simulink model "gps_tracking_both_allsub"  (R2018a)
settings: Solver=VariableStepAuto  StartTime=0.0  StopTime=5*16368/16367600  RelTol=1e-3
libraries: xbsIndex_r4 x171, dspsrcs4 x1
(part 1 of 2)
settings Model: Creator=zhati  LastModifiedBy=Doc_v
settings CodeAppCC: StateflowObjectComments=on
settings SimscapeCC: SimscapeNormalizeSystem=off

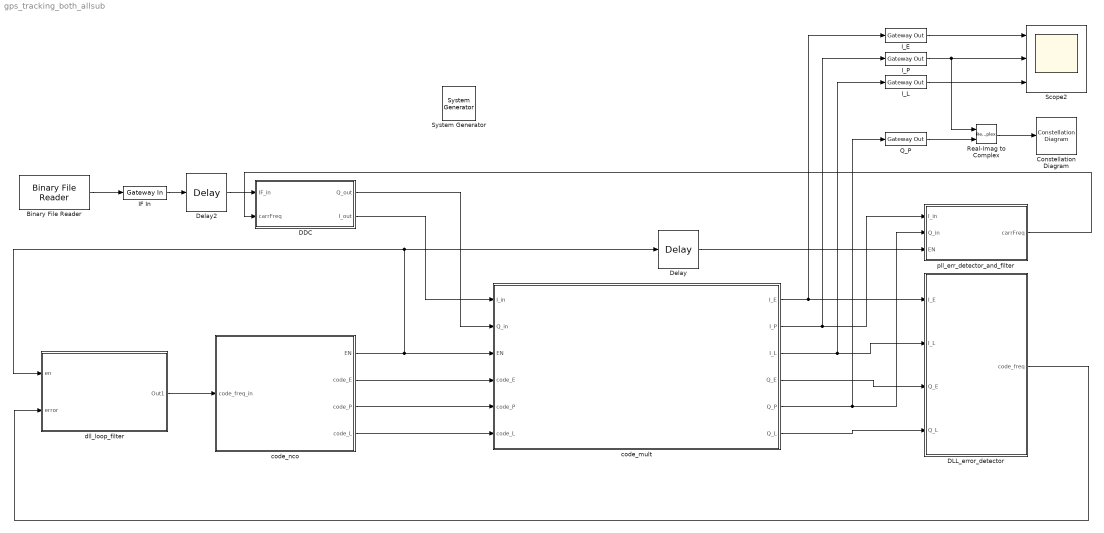
== system gps_tracking_both_allsub ==
  " I_P" : xbsIndex_r4/Gateway Out  inherit_from_input=off  hdl_port=on  rows=1  columns=1  UseAsDAC=off  DACChannel='1'  interface=None  automatic_assignment=on  address_offset=hex2dec('00')  intf_name=''  intf_description=''  timing_constraint=None  locs_specified=off  LOCs={}  io_standard={}  block_type=gatewayout
  " System Generator" : xbsIndex_r4/ System Generator  Tag=genX  xilinxfamily=kintex7  part=xc7k325t  speed=-2  package=ffg900  synthesis_tool=Vivado  clock_wrapper=Clock Enables  directory=./gps_tracking_both_allsub_hwc1  proj_type=Vivado  Synth_file=Vivado Synthesis Defaults  Impl_file=Vivado Implementation Defaults  testbench=on  simulink_period=1/16367600  sysclk_period=10  dcm_input_clock_period=10  incr_netlist=off  trim_vbits=Everywhere in SubSystem  dbl_ovrd=According to Block Masks  core_generation=According to Block Masks  run_coregen=off  deprecated_control=off  eval_field=0  block_type=sysgen
  Binary File Reader : dspsrcs4/Binary File Reader  Filename=E:\sysgen_workspace\gioveAandB_short.bin  HeaderStructure=struct([])  DataType=int8  SamplesPerFrame=1  IsDataComplex=off  NumChannels=1  OutputEOF=off  SampleTime=1/16367600  SimulateUsing=Code generation
      settings: SourceProductName=DSP System Toolbox  SourceProductBaseCode=DS
  Constellation Diagram : ConstellationDiagram
  DDC : Subsystem
  DLL_error_detector : Subsystem
  Delay : xbsIndex_r4/Delay  rst=off  infoeditControl=Selection of Reset will increase slice count due to use of real FFs and instead of SRLs  en=off  latency=1  reg_retiming=off  dbl_ovrd=off  block_type=delay
  Delay2 : xbsIndex_r4/Delay  rst=off  infoeditControl=Selection of Reset will increase slice count due to use of real FFs and instead of SRLs  en=off  latency=1312+28  reg_retiming=off  dbl_ovrd=off  block_type=delay
  IF In : xbsIndex_r4/Gateway In  gui_display_data_type=Fixed-point  arith_type="Signed  (2's comp)"  n_bits=3  bin_pt=0  preci_type=Single  exp_width=8  frac_width=24  rows=1  columns=1  quantization="Round  (unbiased: +/- Inf)"  overflow=Flag as error  period=1/16367600  UseAsADC=off  ADCChannel='1'  interface=None  automatic_assignment=on  address_offset=hex2dec('00')  intf_name=''  intf_description=''  default_value=0  timing_constraint=None  locs_specified=off  LOCs={}  io_standard={}  inherit_from_input=off  hdl_port=on  dbl_ovrd=off  block_type=gatewayin
  I_E : xbsIndex_r4/Gateway Out  inherit_from_input=off  hdl_port=on  rows=1  columns=1  UseAsDAC=off  DACChannel='1'  interface=None  automatic_assignment=on  address_offset=hex2dec('00')  intf_name=''  intf_description=''  timing_constraint=None  locs_specified=off  LOCs={}  io_standard={}  block_type=gatewayout
  I_L : xbsIndex_r4/Gateway Out  inherit_from_input=off  hdl_port=on  rows=1  columns=1  UseAsDAC=off  DACChannel='1'  interface=None  automatic_assignment=on  address_offset=hex2dec('00')  intf_name=''  intf_description=''  timing_constraint=None  locs_specified=off  LOCs={}  io_standard={}  block_type=gatewayout
  Q_P : xbsIndex_r4/Gateway Out  inherit_from_input=off  hdl_port=on  rows=1  columns=1  UseAsDAC=off  DACChannel='1'  interface=None  automatic_assignment=on  address_offset=hex2dec('00')  intf_name=''  intf_description=''  timing_constraint=None  locs_specified=off  LOCs={}  io_standard={}  block_type=gatewayout
  Real-Imag to Complex : RealImagToComplex
  Scope2 : Scope  NumInputPorts=3
  code_mult : Subsystem
  code_nco : Subsystem
  dll_loop_filter : Subsystem
  pll_err_detector_and_filter : Subsystem
  wires:
  Binary File Reader/1 -> IF In/1
  IF In/1 -> Delay2/1
  DLL_error_detector/1(code_freq) -> dll_loop_filter/2(error)
  dll_loop_filter/1(Out1) -> code_nco/1(code_freq_in)
  Delay2/1 -> DDC/1(IF_in)
  code_nco/2(code_E) -> code_mult/4(code_E)
  code_nco/3(code_P) -> code_mult/5(code_P)
  code_nco/4(code_L) -> code_mult/6(code_L)
  code_mult/1(I_E) -> I_E/1, DLL_error_detector/1(I_E)
  code_mult/3(I_L) -> I_L/1, DLL_error_detector/2(I_L)
  code_mult/4(Q_E) -> DLL_error_detector/3(Q_E)
  code_mult/6(Q_L) -> DLL_error_detector/4(Q_L)
  code_nco/1(EN) -> dll_loop_filter/1(en), Delay/1, code_mult/3(EN)
  DDC/2(I_out) -> code_mult/1(I_in)
  DDC/1(Q_out) -> code_mult/2(Q_in)
  code_mult/2(I_P) -> pll_err_detector_and_filter/1(I_in), " I_P"/1
  code_mult/5(Q_P) -> Q_P/1, pll_err_detector_and_filter/2(Q_in)
  Delay/1 -> pll_err_detector_and_filter/3(EN)
  pll_err_detector_and_filter/1(carrFreq) -> DDC/2(carrFreq)
  I_E/1 -> Scope2/1
  " I_P"/1 -> Real-Imag to Complex/1, Scope2/2
  I_L/1 -> Scope2/3
  Q_P/1 -> Real-Imag to Complex/2
  Real-Imag to Complex/1 -> Constellation Diagram/1

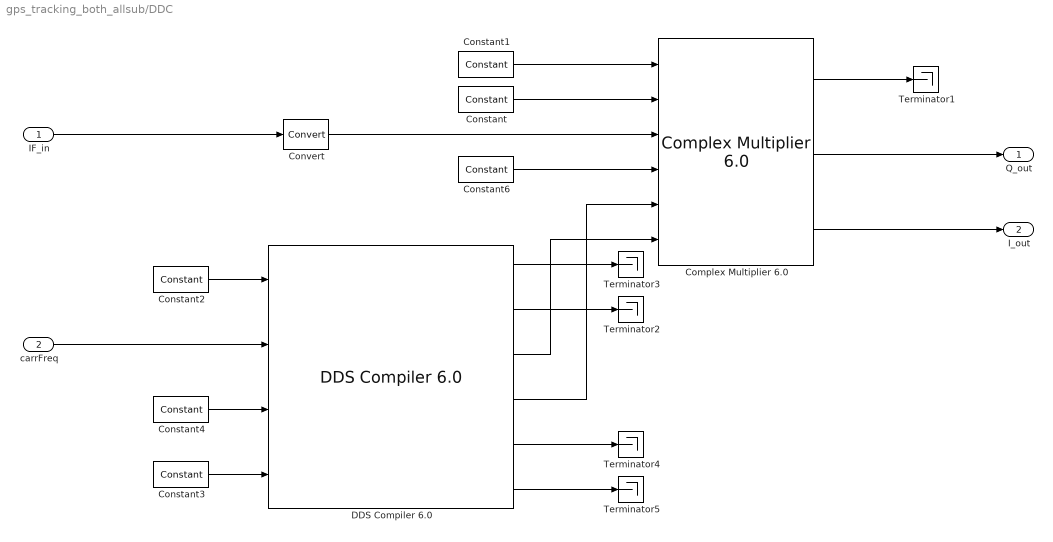
== system gps_tracking_both_allsub/DDC ==
  IF_in : Inport
  carrFreq : Inport  Port=2
  "Complex Multiplier 6.0 " : xbsIndex_r4/Complex Multiplier 6.0   hasatlast=off  hasatuser=off  atuserwidth=1  hasbtlast=off  hasbtuser=off  btuserwidth=1  multtype=Use_Mults  optimizegoal=Resources  flowcontrol=NonBlocking  outputwidth=19  roundmode=Truncate  hasctrltlast=off  hasctrltuser=off  ctrltuserwidth=1  outtlastbehv=Null  latencyconfig=Automatic  minimumlatency=37  aclken=off  aresetn=off  trim_axipin_name=on  simulation_type=hybrid_sim  simulation_model=sysgen:cmpy_v6_0  data_path_portlist={ 's_axis_a_tdata_real', 's_axis_a_tdata_imag', 's_axis_b_tdata_real', 's_axis_b_tdata_imag', 's_axis_ctrl_tdata_rounding_bit', 'm_axis_dout_tdata_real', 'm_axis_dout_tdata_imag' }  aportwidth=63  bportwidth=63  ip_name=Complex Multiplier  ip_version=6.0  dsptool_ready=true  ipcore_usecache=true  ipcore_useipmodelcache=true  ipcore_verbose=false  ipcore_latency_parameter='minimumlatency'  wrapper_available=true  port_translation_map={ 'aclken' => 'en', 'aresetn' => 'rst'}  block_type=cmpy_v6_0
  Constant : xbsIndex_r4/Constant  const=0  gui_display_data_type=Fixed-point  arith_type=Signed (2's comp)  n_bits=16  bin_pt=13  preci_type=Single  exp_width=8  frac_width=24  explicit_period=on  period=1/16367600  equ=P=C  opselect=C  inp2=PCIN>>17  opr=+  inp1=P  carry=CIN  dbl_ovrd=off  block_type=constant
  Constant{1..4,6} (5 alike) : xbsIndex_r4/Constant  const=1  gui_display_data_type=Boolean  arith_type=Boolean  n_bits=16  bin_pt=14  preci_type=Single  exp_width=8  frac_width=24  explicit_period=on  period=1/16367600  equ=P=C  opselect=C  inp2=PCIN>>17  opr=+  inp1=P  carry=CIN  dbl_ovrd=off  block_type=constant
  Convert : xbsIndex_r4/Convert  gui_display_data_type=Fixed-point  arith_type="Signed  (2's comp)"  n_bits=16  bin_pt=13  float_type=Single  exp_bits=8  fraction_bits=24  quantization=Truncate  overflow=Wrap  en=off  latency=1  pipeline=off  dbl_ovrd=off  block_type=convert
  "DDS Compiler 6.0 " : xbsIndex_r4/DDS Compiler 6.0   partspresent=Phase_Generator_and_SIN_COS_LUT  dds_clock_rate=100  channels=1  mode_of_operation=Standard  modulus=9  parameter_entry=Hardware_Parameters  spurious_free_dynamic_range=45  frequency_resolution=0.4  noise_shaping=None  phase_width=24  output_width=16  output_selection=Sine_and_Cosine  negative_sine=off  negative_cosine=off  amplitude_mode=Full_Range  memory_type=Auto  optimization_goal=Auto  dsp48_use=Minimal  resync=off  latency_configuration=Auto  latency=1  has_phase_out=on  has_aclken=off  has_aresetn=off  explicit_period=off  period=1  data_has_tlast=Not_Required  has_tready=on  s_phase_has_tuser=Not_Required  m_data_has_tuser=Not_Required  m_phase_has_tuser=Not_Required  s_phase_tuser_width=1  output_form=Twos_Complement  s_config_sync_mode=On_Vector  phase_increment=Streaming  output_frequency1=0  output_frequency2=0  output_frequency3=0  output_frequency4=0  output_frequency5=0  output_frequency6=0  output_frequency7=0  output_frequency8=0  output_frequency9=0  output_frequency10=0  output_frequency11=0  output_frequency12=0  output_frequency13=0  output_frequency14=0  output_frequency15=0  output_frequency16=0  pinc1='0'  pinc2='0'  pinc3='0'  pinc4='0'  pinc5='0'  pinc6='0'  pinc7='0'  pinc8='0'  pinc9='0'  pinc10='0'  pinc11='0'  pinc12='0'  pinc13='0'  pinc14='0'  pinc15='0'  pinc16='0'  phase_offset=None  phase_offset_angles1=0  phase_offset_angles2=0  phase_offset_angles3=0  phase_offset_angles4=0  phase_offset_angles5=0  phase_offset_angles6=0  phase_offset_angles7=0  phase_offset_angles8=0  phase_offset_angles9=0  phase_offset_angles10=0  phase_offset_angles11=0  phase_offset_angles12=0  phase_offset_angles13=0  phase_offset_angles14=0  phase_offset_angles15=0  phase_offset_angles16=0  poff1='0'  poff2='0'  poff3='0'  poff4='0'  poff5='0'  poff6='0'  poff7='0'  poff8='0'  poff9='0'  poff10='0'  poff11='0'  poff12='0'  poff13='0'  poff14='0'  poff15='0'  poff16='0'  trim_axipin_name=on  simulation_type=hybrid_sim  simulation_model=sysgen:xddsv6_0_cmodel  data_path_portlist={ 's_axis_config_tdata_poff', 's_axis_config_tdata_chan0_poff', 's_axis_config_tdata_pinc', 's_axis_config_tdata_chan0_pinc', 's_axis_phase_tdata_resync', 's_axis_phase_tdata_chan0_resync', 's_axis_phase_tdata_poff', 's_axis_phase_tdata_chan0_poff', 's_axis_phase_tdata_pinc', 's_axis_phase_tdata_chan0_pinc', 's_axis_phase_tdata_phase_in', 'm_axis_data_tdata_sine', 'm_axis_data_tdata_chan0_sine', 'm_axis_data_tdata_cosine', 'm_axis_data_tdata_chan0_cosine', 'm_axis_phase_tdata_phase_out', 'm_axis_phase_tdata_chan0_phase_out'}  por_mode=false  gui_behaviour=Sysgen  ip_name=DDS Compiler  ip_version=6.0  dsptool_ready=true  wrapper_available=true  port_translation_map={ 'aclken' => 'en', 'aresetn' => 'rst' }  ipcore_usecache=true  ipcore_useipmodelcache=true  ipcore_xco_need_fpga_part=true  ipcore_verbose=false  block_type=dds_compiler_v6_0
  Terminator{1..5} (5 alike) : Terminator
  Q_out : Outport
  I_out : Outport  Port=2
  wires:
  "DDS Compiler 6.0 "/6 -> Terminator5/1
  "DDS Compiler 6.0 "/5 -> Terminator4/1
  "DDS Compiler 6.0 "/1 -> Terminator3/1
  "DDS Compiler 6.0 "/2 -> Terminator2/1
  carrFreq/1 -> "DDS Compiler 6.0 "/2
  "Complex Multiplier 6.0 "/3 -> I_out/1
  Constant6/1 -> "Complex Multiplier 6.0 "/4
  Constant3/1 -> "DDS Compiler 6.0 "/4
  Constant/1 -> "Complex Multiplier 6.0 "/2
  "Complex Multiplier 6.0 "/1 -> Terminator1/1
  IF_in/1 -> Convert/1
  "DDS Compiler 6.0 "/3 -> "Complex Multiplier 6.0 "/6
  Constant2/1 -> "DDS Compiler 6.0 "/1
  "Complex Multiplier 6.0 "/2 -> Q_out/1
  Constant1/1 -> "Complex Multiplier 6.0 "/1
  "DDS Compiler 6.0 "/4 -> "Complex Multiplier 6.0 "/5
  Constant4/1 -> "DDS Compiler 6.0 "/3
  Convert/1 -> "Complex Multiplier 6.0 "/3

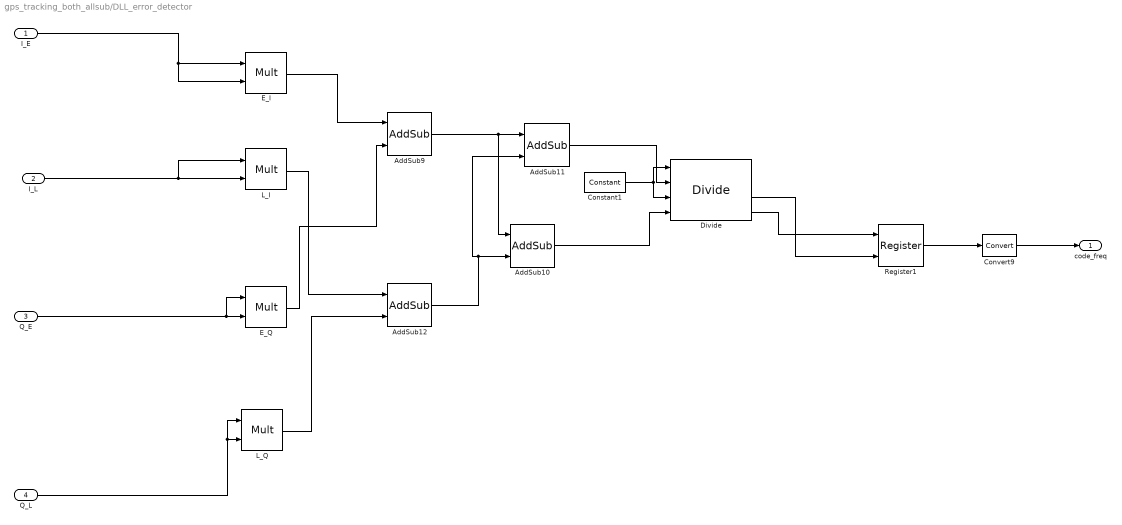
== system gps_tracking_both_allsub/DLL_error_detector ==
  I_E : Inport
  I_L : Inport  Port=2
  Q_E : Inport  Port=3
  Q_L : Inport  Port=4
  AddSub10 : xbsIndex_r4/AddSub  mode=Addition  use_carryin=off  use_carryout=off  en=off  latency=1  precision=User Defined  arith_type="Signed  (2's comp)"  n_bits=35  bin_pt=0  quantization=Truncate  overflow=Flag as error  use_behavioral_HDL=off  hw_selection=Fabric  pipelined=off  dbl_ovrd=off  block_type=addsub
  AddSub11 : xbsIndex_r4/AddSub  mode=Subtraction  use_carryin=off  use_carryout=off  en=off  latency=1  precision=User Defined  arith_type="Signed  (2's comp)"  n_bits=35  bin_pt=0  quantization=Truncate  overflow=Flag as error  use_behavioral_HDL=off  hw_selection=Fabric  pipelined=off  dbl_ovrd=off  block_type=addsub
  AddSub12 : xbsIndex_r4/AddSub  mode=Addition  use_carryin=off  use_carryout=off  en=off  latency=1  precision=Full  arith_type="Signed  (2's comp)"  n_bits=16  bin_pt=15  quantization=Truncate  overflow=Wrap  use_behavioral_HDL=off  hw_selection=Fabric  pipelined=off  dbl_ovrd=off  block_type=addsub
  AddSub9 : xbsIndex_r4/AddSub  mode=Addition  use_carryin=off  use_carryout=off  en=off  latency=1  precision=Full  arith_type="Signed  (2's comp)"  n_bits=16  bin_pt=15  quantization=Truncate  overflow=Wrap  use_behavioral_HDL=off  hw_selection=Fabric  pipelined=off  dbl_ovrd=off  block_type=addsub
  Constant1 : xbsIndex_r4/Constant  const=1.0  gui_display_data_type=Boolean  arith_type=Boolean  n_bits=16  bin_pt=14  preci_type=Single  exp_width=8  frac_width=24  explicit_period=off  period=1  equ=P=C  opselect=C  inp2=PCIN>>17  opr=+  inp1=P  carry=CIN  dbl_ovrd=off  block_type=constant
  Convert9 : xbsIndex_r4/Convert  gui_display_data_type=Fixed-point  arith_type="Signed  (2's comp)"  n_bits=16  bin_pt=14  float_type=Single  exp_bits=8  fraction_bits=24  quantization=Truncate  overflow=Saturate  en=off  latency=1  pipeline=off  dbl_ovrd=off  block_type=convert
  Divide : xbsIndex_r4/Divide  flow_control=Blocking  axi_optimize_goal=Resources  algorithm_type=High_Radix  infoedit1=Specify output fraction-width for Fixed-point division.  fractional_width=14  infoedit2=Specify latency for Floating-point division.  latency=1  rate=1  has_a_tlast=off  has_a_tuser=off  has_b_tlast=off  has_b_tuser=off  en=off  has_result_tready=off  result_tlast_behv=Pass_A_TLAST  has_underflow=off  has_overflow=off  has_invalid_op=off  has_divide_by_zero=off  fpo_op_type=mergeddivide  block_type=divide
      settings: infoedit=Blocking: Wait for data on all inputs, allow back-pressure.<br>NonBlocking: operate every cycle in which all inputs are valid, no back-pressure.
  E_I : xbsIndex_r4/Mult  precision=Full  arith_type="Signed  (2's comp)"  n_bits=16  bin_pt=14  quantization=Truncate  overflow=Wrap  en=off  latency=1  use_behavioral_HDL=off  opt=Speed  use_embedded=on  optimum_pipeline=off  pipeline=on  dbl_ovrd=off  use_rpm=on  placement_style=Triangular  block_type=mult
  E_Q : xbsIndex_r4/Mult  precision=Full  arith_type="Signed  (2's comp)"  n_bits=16  bin_pt=14  quantization=Truncate  overflow=Wrap  en=off  latency=1  use_behavioral_HDL=off  opt=Speed  use_embedded=on  optimum_pipeline=off  pipeline=on  dbl_ovrd=off  use_rpm=on  placement_style=Triangular  block_type=mult
  L_I : xbsIndex_r4/Mult  precision=Full  arith_type="Signed  (2's comp)"  n_bits=16  bin_pt=14  quantization=Truncate  overflow=Wrap  en=off  latency=1  use_behavioral_HDL=off  opt=Speed  use_embedded=on  optimum_pipeline=off  pipeline=on  dbl_ovrd=off  use_rpm=on  placement_style=Triangular  block_type=mult
  L_Q : xbsIndex_r4/Mult  precision=Full  arith_type="Signed  (2's comp)"  n_bits=16  bin_pt=14  quantization=Truncate  overflow=Wrap  en=off  latency=1  use_behavioral_HDL=off  opt=Speed  use_embedded=on  optimum_pipeline=off  pipeline=on  dbl_ovrd=off  use_rpm=on  placement_style=Triangular  block_type=mult
  Register1 : xbsIndex_r4/Register  init=0  rst=off  en=on  dbl_ovrd=off  block_type=register
  code_freq : Outport
  wires:
  AddSub9/1 -> AddSub11/1, AddSub10/1
  I_L/1 -> L_I/1, L_I/2
  AddSub12/1 -> AddSub10/2, AddSub11/2
  Q_L/1 -> L_Q/1, L_Q/2
  Q_E/1 -> E_Q/1, E_Q/2
  Divide/4 -> Register1/1
  AddSub11/1 -> Divide/2
  AddSub10/1 -> Divide/4
  Constant1/1 -> Divide/1, Divide/3
  L_I/1 -> AddSub12/1
  Divide/3 -> Register1/2
  E_Q/1 -> AddSub9/2
  E_I/1 -> AddSub9/1
  Register1/1 -> Convert9/1
  L_Q/1 -> AddSub12/2
  I_E/1 -> E_I/2, E_I/1
  Convert9/1 -> code_freq/1

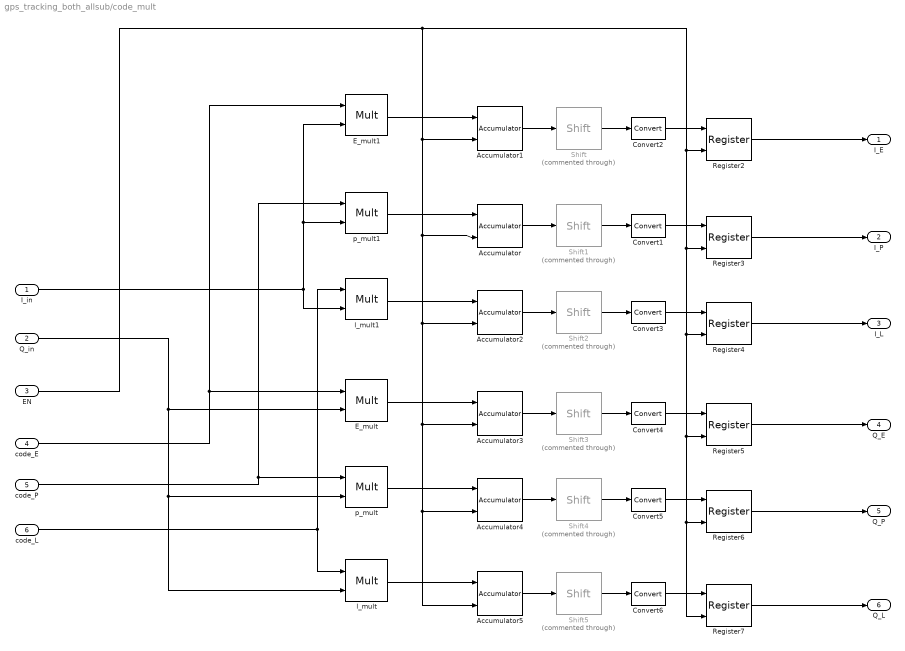
== system gps_tracking_both_allsub/code_mult ==
  I_in : Inport
  Q_in : Inport  Port=2
  EN : Inport  Port=3
  code_E : Inport  Port=4
  code_P : Inport  Port=5
  code_L : Inport  Port=6
  Accumulator{,1,3..5} (5 alike) : xbsIndex_r4/Accumulator  operation=Add  n_bits=30  overflow=Wrap  scale=1  rst=on  hasbypass=off  infoeditControl=reset for floating point data type must be asserted for a minimum of 2 cycles  en=off  latency=1  msb_inp=100  msb=100  lsb=-100  use_behavioral_HDL=on  implementation=Fabric  dbl_ovrd=off  block_type=accum
  Accumulator2 : xbsIndex_r4/Accumulator  operation=Add  n_bits=32  overflow=Wrap  scale=1  rst=on  hasbypass=off  infoeditControl=reset for floating point data type must be asserted for a minimum of 2 cycles  en=off  latency=1  msb_inp=100  msb=100  lsb=-100  use_behavioral_HDL=on  implementation=Fabric  dbl_ovrd=off  block_type=accum
  Convert{1..6} (6 alike) : xbsIndex_r4/Convert  gui_display_data_type=Fixed-point  arith_type="Signed  (2's comp)"  n_bits=16  bin_pt=0  float_type=Single  exp_bits=8  fraction_bits=24  quantization=Truncate  overflow=Flag as error  en=off  latency=1  pipeline=off  dbl_ovrd=off  block_type=convert
  E_mult : xbsIndex_r4/Mult  precision=Full  arith_type="Signed  (2's comp)"  n_bits=16  bin_pt=14  quantization=Truncate  overflow=Wrap  en=off  latency=1  use_behavioral_HDL=off  opt=Speed  use_embedded=on  optimum_pipeline=off  pipeline=on  dbl_ovrd=off  use_rpm=on  placement_style=Triangular  block_type=mult
  E_mult1 : xbsIndex_r4/Mult  precision=Full  arith_type="Signed  (2's comp)"  n_bits=16  bin_pt=14  quantization=Truncate  overflow=Wrap  en=off  latency=1  use_behavioral_HDL=off  opt=Speed  use_embedded=on  optimum_pipeline=off  pipeline=on  dbl_ovrd=off  use_rpm=on  placement_style=Triangular  block_type=mult
  Register{2..7} (6 alike) : xbsIndex_r4/Register  init=0  rst=off  en=on  dbl_ovrd=off  block_type=register
  Shift{,1..5} (6 alike) : xbsIndex_r4/Shift  Commented=through  shift_dir=Right  shift_bits=16  en=off  latency=1  precision=Full  arith_type="Signed  (2's comp)"  n_bits=16  bin_pt=14  quantization=Truncate  overflow=Wrap  dbl_ovrd=off  block_type=shift
  l_mult : xbsIndex_r4/Mult  precision=Full  arith_type="Signed  (2's comp)"  n_bits=16  bin_pt=14  quantization=Truncate  overflow=Wrap  en=off  latency=1  use_behavioral_HDL=off  opt=Speed  use_embedded=on  optimum_pipeline=off  pipeline=on  dbl_ovrd=off  use_rpm=on  placement_style=Triangular  block_type=mult
  l_mult1 : xbsIndex_r4/Mult  precision=Full  arith_type="Signed  (2's comp)"  n_bits=16  bin_pt=14  quantization=Truncate  overflow=Wrap  en=off  latency=1  use_behavioral_HDL=off  opt=Speed  use_embedded=on  optimum_pipeline=off  pipeline=on  dbl_ovrd=off  use_rpm=on  placement_style=Triangular  block_type=mult
  p_mult : xbsIndex_r4/Mult  precision=Full  arith_type="Signed  (2's comp)"  n_bits=16  bin_pt=14  quantization=Truncate  overflow=Wrap  en=off  latency=1  use_behavioral_HDL=off  opt=Speed  use_embedded=on  optimum_pipeline=off  pipeline=on  dbl_ovrd=off  use_rpm=on  placement_style=Triangular  block_type=mult
  p_mult1 : xbsIndex_r4/Mult  precision=Full  arith_type="Signed  (2's comp)"  n_bits=16  bin_pt=14  quantization=Truncate  overflow=Wrap  en=off  latency=1  use_behavioral_HDL=off  opt=Speed  use_embedded=on  optimum_pipeline=off  pipeline=on  dbl_ovrd=off  use_rpm=on  placement_style=Triangular  block_type=mult
  I_E : Outport
  I_P : Outport  Port=2
  I_L : Outport  Port=3
  Q_E : Outport  Port=4
  Q_P : Outport  Port=5
  Q_L : Outport  Port=6
  wires:
  Register7/1 -> Q_L/1
  Register3/1 -> I_P/1
  Q_in/1 -> l_mult/2, p_mult/2, E_mult/2
  l_mult1/1 -> Accumulator2/1
  code_E/1 -> E_mult1/1, E_mult/1
  I_in/1 -> E_mult1/2, p_mult1/2, l_mult1/2
  Shift3/1 -> Convert4/1
  Convert3/1 -> Register4/1
  code_P/1 -> p_mult1/1, p_mult/1
  Accumulator2/1 -> Shift2/1
  Shift4/1 -> Convert5/1
  Shift5/1 -> Convert6/1
  EN/1 -> Register3/2, Register4/2, Register5/2, Register6/2, Register7/2, Register2/2, Accumulator2/2, Accumulator3/2, Accumulator4/2, Accumulator5/2, Accumulator/2, Accumulator1/2
  Accumulator1/1 -> Shift/1
  Shift2/1 -> Convert3/1
  Shift/1 -> Convert2/1
  p_mult/1 -> Accumulator4/1
  Register5/1 -> Q_E/1
  Accumulator/1 -> Shift1/1
  E_mult/1 -> Accumulator3/1
  Accumulator5/1 -> Shift5/1
  l_mult/1 -> Accumulator5/1
  Shift1/1 -> Convert1/1
  Accumulator3/1 -> Shift3/1
  Convert5/1 -> Register6/1
  Convert4/1 -> Register5/1
  Convert1/1 -> Register3/1
  p_mult1/1 -> Accumulator/1
  Convert2/1 -> Register2/1
  code_L/1 -> l_mult/1, l_mult1/1
  Accumulator4/1 -> Shift4/1
  E_mult1/1 -> Accumulator1/1
  Convert6/1 -> Register7/1
  Register6/1 -> Q_P/1
  Register4/1 -> I_L/1
  Register2/1 -> I_E/1

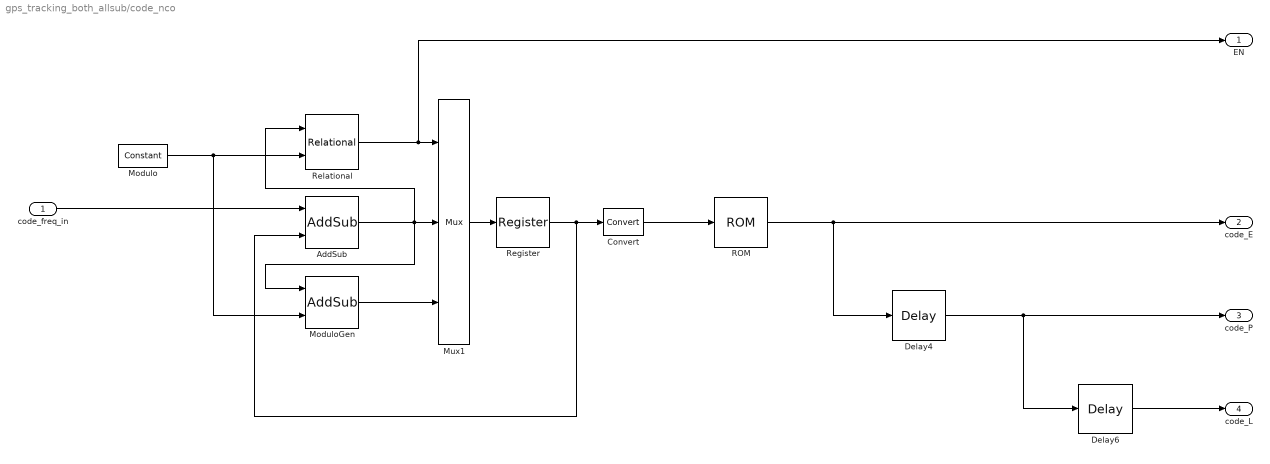
== system gps_tracking_both_allsub/code_nco ==
  code_freq_in : Inport
  AddSub : xbsIndex_r4/AddSub  mode=Addition  use_carryin=off  use_carryout=off  en=off  latency=0  precision=User Defined  arith_type=Unsigned  n_bits=42  bin_pt=32  quantization=Truncate  overflow=Flag as error  use_behavioral_HDL=off  hw_selection=Fabric  pipelined=off  dbl_ovrd=off  block_type=addsub
  Convert : xbsIndex_r4/Convert  gui_display_data_type=Fixed-point  arith_type=Unsigned  n_bits=10  bin_pt=0  float_type=Single  exp_bits=8  fraction_bits=24  quantization=Truncate  overflow=Wrap  en=off  latency=1  pipeline=off  dbl_ovrd=off  block_type=convert
  Delay4 : xbsIndex_r4/Delay  rst=off  infoeditControl=Selection of Reset will increase slice count due to use of real FFs and instead of SRLs  en=off  latency=8  reg_retiming=off  dbl_ovrd=off  block_type=delay
  Delay6 : xbsIndex_r4/Delay  rst=off  infoeditControl=Selection of Reset will increase slice count due to use of real FFs and instead of SRLs  en=off  latency=8  reg_retiming=off  dbl_ovrd=off  block_type=delay
  Modulo : xbsIndex_r4/Constant  const=1023-2e-32  gui_display_data_type=Fixed-point  arith_type=Unsigned  n_bits=42  bin_pt=32  preci_type=Single  exp_width=8  frac_width=24  explicit_period=on  period=1/16367600  equ=P=C  opselect=C  inp2=PCIN>>17  opr=+  inp1=P  carry=CIN  dbl_ovrd=off  block_type=constant
  ModuloGen : xbsIndex_r4/AddSub  mode=Subtraction  use_carryin=off  use_carryout=off  en=off  latency=0  precision=User Defined  arith_type=Unsigned  n_bits=42  bin_pt=32  quantization=Truncate  overflow=Wrap  use_behavioral_HDL=off  hw_selection=Fabric  pipelined=off  dbl_ovrd=off  block_type=addsub
  Mux1 : xbsIndex_r4/Mux  inputs=2  en=off  latency=0  precision=Full  arith_type=Unsigned  n_bits=16  bin_pt=14  quantization=Truncate  overflow=Wrap  dbl_ovrd=off  block_type=mux
  ROM : xbsIndex_r4/ROM  depth=1023  initVector=[1,1,1,1,1,1,-1,-1,1,1,1,-1,-1,1,-1,1,-1,-1,1,-1,1,-1,-1,1,-1,-1,-1,-1,1,-1,-1,-1,1,1,-1,-1,1,-1,-1,1,-1,-1,1,-1,1,-1,-1,-1,-1,-1,1,-1,1,-1,-1,-1,1,-1,-1,1,1,-1,1,-1,-1,1,1,-1,-1,1,1,-1,1,-1,-1,1,1,1,1,1,-1,1,1,1,1,1,-1,1,1,-1,-1,1,1,-1,1,-1,1,1,1,1,1,-1,1,-1,-1,1,1,1,1,1,1,1,1,-1,-1,1,1,1,1,1,-1,1,-1,-1,1,1,-1,1,1,1,-1,-1,1,-1,1,-1,-1,-1,1,-1,1,-1,1,1,-1,-1,1,-1,-1,-1,1,-1,1,-1,1,1,1,-1,1,1,1,1,1,1,-1,-1,1,1,1,-1,-1,1,1,1,1,1,-1,-1,-1,1,1,1,-1,1,-1,1,1,1,1,-1,-1,1,1,-1,1,1,1,1,-1,-1,-1,-1,1,1,1,-1,1,1,1,1,1,-1,-1,1,-1,1,1,-1,1,-1,1,1,1,-1,-1,-1,1,1,1,-1,1,-1,1,-1,1,-1,1,-1,-1,-1,-1,-1,1,-1,-1,1,-1,1,1,-1,-1,1,-1,1,-1,1,-1,1,1,1,1,-1,-1,-1,-1,-1,-1,-1,1,1,1,1,-1,1,1,1,-1,1,1,-1,-1,-1,1,-1,1,1,1,1,1,1,-1,1,-1,-1,1,-1,-1,-1,1,1,-1,1,1,1,-1,-1,1,-1,-1,-1,-1,1,-1,1,-1,-1,-1,-1,-1,-1,-1,-1,-1,1,-1,-1,1,1,-1,1,1,1,1,-1,-1,-1,1,1,1,1,1,-1,1,-1,-1,1,-1,1,1,1,1,-1,-1,-1,1,1,1,1,1,1,1,1,-1,1,-1,1,-1,-1,-1,-1,-1,1,1,1,-1,1,-1,-1,-1,1,-1,1,-1,1,1,-1,1,-1,1,-1,-1,-1,-1,1,1,-1,-1,1,-1,-1,-1,1,1,1,1,-1,-1,-1,1,1,1,1,1,-1,-1,1,1,1,1,1,1,-1,-1,1,-1,-1,-1,1,1,1,1,-1,-1,1,1,1,-1,1,-1,-1,1,1,-1,-1,-1,1,1,-1,-1,-1,1,-1,-1,1,1,-1,-1,1,1,-1,1,-1,-1,-1,1,1,-1,1,1,1,-1,1,-1,-1,1,1,1,-1,-1,-1,-1,-1,1,-1,1,-1,-1,-1,-1,1,1,1,-1,-1,-1,-1,-1,1,-1,-1,1,-1,1,1,-1,-1,1,1,-1,-1,1,-1,-1,-1,-1,1,-1,1,-1,1,1,-1,1,1,1,1,1,-1,1,-1,1,-1,-1,1,1,-1,1,1,-1,-1,1,-1,1,1,1,-1,-1,1,1,-1,-1,1,1,-1,-1,-1,1,-1,-1,-1,-1,1,-1,1,1,-1,-1,-1,1,1,1,-1,1,1,-1,-1,-1,1,-1,-1,-1,-1,1,1,-1,1,-1,-1,-1,1,-1,-1,-1,-1,-1,1,-1,1,1,-1,-1,1,1,1,-1,-1,1,-1,-1,1,1,-1,-1,1,1,-1,1,1,1,-1,-1,-1,1,-1,-1,-1,1,1,-1,1,1,1,1,1,-1,1,-1,-1,1,1,1,-1,-1,-1,1,-1,-1,-1,-1,-1,-1,1,1,1,1,-1,-1,1,-1,1,1,-1,1,-1,-1,1,-1,-1,1,-1,1,-1,-1,-1,1,1,1,1,1,1,-1,1,1,-1,1,1,-1,1,1,1,-1,-1,1,-1,-1,-1,1,-1,1,1,-1,1,-1,-1,1,1,1,-1,-1,-1,1,-1,1,1,-1,1,1,-1,1,-1,1,1,1,-1,-1,1,1,1,-1,1,-1,-1,1,-1,-1,1,-1,-1,-1,-1,-1,1,-1,1,-1,1,-1,1,1,1,1,-1,-1,1,1,-1,1,-1,-1,-1,-1,-1,-1,1,-1,1,1,1,1,-1,-1,1,-1,1,-1,1,-1,-1,-1,1,1,-1,-1,-1,1,-1,1,-1,1,1,1,-1,1,1,-1,1,-1,1,-1,-1,1,-1,-1,1,-1,1,-1,1,1,-1,-1,1,1,-1,1,1,-1,1,-1,-1,1,-1,1,1,1,-1,-1,-1,1,-1,1,1,-1,-1,1,-1,1,1,-1,-1,1,-1,1,-1,-1,1,-1,1,-1,1,1,1,-1,1,1,1,-1,1,1,-1,1,-1,1,-1,1,-1,1,-1,1,-1,1,1,-1,1,-1,1,1,-1,-1,1,-1,1,-1,1,-1,-1,1,-1,-1,-1,1,1,-1,1,-1,1,-1,-1,1,-1,1,-1,-1,1,-1,1,-1,-1,1,-1,-1,1,1,1,-1,-1,1,-1,-1,-1,-1,-1,-1,1,-1,-1,1,1,-1,1,-1,-1,-1,1,-1,1,1,1,1,-1,1,1,-1,1,1,-1,-1,1,-1,-1,-1,-1,1,1,1,-1,1,-1,1,-1,1,-1,-1,1,1,-1,1,-1,-1,1,-1,-1,1,-1,1,-1,-1,-1,-1,1,-1,-1,-1,1,1,-1,-1,-1,1,-1,-1,-1,1,-1,1,-1,-1,-1,1,-1,1,1,-1,1,-1,1,1,-1,1,-1,-1,-1,1,1,1,1,1,1,-1,-1,-1,1,-1]  distributed_mem=Block RAM  rst=off  init_reg=0  en=off  latency=1  gui_display_data_type=Fixed-point  arith_type="Signed  (2's comp)"  n_bits=2  bin_pt=0  preci_type=Single  exp_width=8  frac_width=24  optimize=Area  use_rpm=on  dbl_ovrd=off  block_type=sprom
  Register : xbsIndex_r4/Register  init=0  rst=off  en=off  dbl_ovrd=off  block_type=register
  Relational : xbsIndex_r4/Relational  mode=a>=b  op_type=Bool  en=off  latency=0  dbl_ovrd=off  block_type=relational
  EN : Outport
  code_E : Outport  Port=2
  code_P : Outport  Port=3
  code_L : Outport  Port=4
  wires:
  AddSub/1 -> ModuloGen/1, Relational/1, Mux1/2
  ROM/1 -> Delay4/1, code_E/1
  Relational/1 -> EN/1, Mux1/1
  Register/1 -> Convert/1, AddSub/2
  Mux1/1 -> Register/1
  Modulo/1 -> ModuloGen/2, Relational/2
  ModuloGen/1 -> Mux1/3
  code_freq_in/1 -> AddSub/1
  Convert/1 -> ROM/1
  Delay4/1 -> Delay6/1, code_P/1
  Delay6/1 -> code_L/1

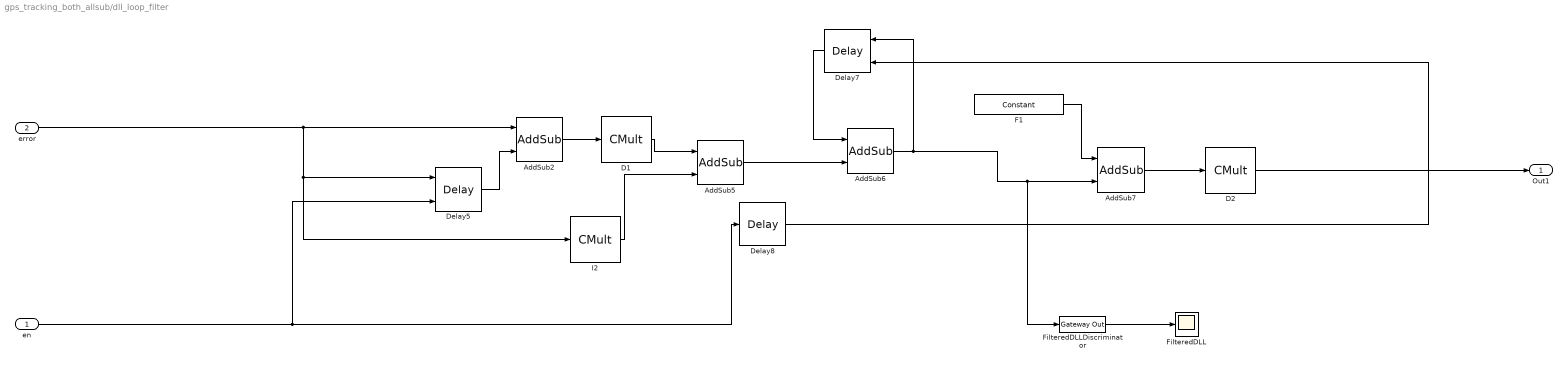
== system gps_tracking_both_allsub/dll_loop_filter ==
  en : Inport
  error : Inport  Port=2
  AddSub2 : xbsIndex_r4/AddSub  mode=Subtraction  use_carryin=off  use_carryout=off  en=off  latency=1  precision=Full  arith_type="Signed  (2's comp)"  n_bits=16  bin_pt=15  quantization=Truncate  overflow=Wrap  use_behavioral_HDL=off  hw_selection=Fabric  pipelined=off  dbl_ovrd=off  block_type=addsub
  AddSub5 : xbsIndex_r4/AddSub  mode=Addition  use_carryin=off  use_carryout=off  en=off  latency=1  precision=Full  arith_type="Signed  (2's comp)"  n_bits=16  bin_pt=15  quantization=Truncate  overflow=Wrap  use_behavioral_HDL=off  hw_selection=Fabric  pipelined=off  dbl_ovrd=off  block_type=addsub
  AddSub6 : xbsIndex_r4/AddSub  mode=Addition  use_carryin=off  use_carryout=off  en=off  latency=1  precision=User Defined  arith_type="Signed  (2's comp)"  n_bits=32  bin_pt=15  quantization=Truncate  overflow=Flag as error  use_behavioral_HDL=off  hw_selection=Fabric  pipelined=off  dbl_ovrd=off  block_type=addsub
  AddSub7 : xbsIndex_r4/AddSub  mode=Addition  use_carryin=off  use_carryout=off  en=off  latency=1  precision=Full  arith_type="Signed  (2's comp)"  n_bits=16  bin_pt=15  quantization=Truncate  overflow=Wrap  use_behavioral_HDL=off  hw_selection=Fabric  pipelined=off  dbl_ovrd=off  block_type=addsub
  D1 : xbsIndex_r4/CMult  const=5.297297  gui_display_data_type=Fixed-point  const_n_bits=20  const_bin_pt=15  float_type=Single  exp_bits=8  fraction_bits=24  en=off  latency=1  precision=Full  arith_type="Signed  (2's comp)"  n_bits=16  bin_pt=14  quantization=Truncate  overflow=Wrap  use_behavioral_HDL=off  mem_type=Distributed RAM  pipeline=off  dbl_ovrd=off  block_type=cmult
  D2 : xbsIndex_r4/CMult  const=1/16367600  gui_display_data_type=Fixed-point  const_n_bits=48  const_bin_pt=48  float_type=Single  exp_bits=8  fraction_bits=24  en=off  latency=1  precision=User Defined  arith_type="Signed  (2's comp)"  n_bits=32  bin_pt=32  quantization=Truncate  overflow=Flag as error  use_behavioral_HDL=off  mem_type=Distributed RAM  pipeline=off  dbl_ovrd=off  block_type=cmult
  Delay5 : xbsIndex_r4/Delay  rst=off  infoeditControl=Selection of Reset will increase slice count due to use of real FFs and instead of SRLs  en=on  latency=1  reg_retiming=off  dbl_ovrd=off  block_type=delay
  Delay7 : xbsIndex_r4/Delay  rst=off  infoeditControl=Selection of Reset will increase slice count due to use of real FFs and instead of SRLs  en=on  latency=1  reg_retiming=off  dbl_ovrd=off  block_type=delay
  Delay8 : xbsIndex_r4/Delay  rst=off  infoeditControl=Selection of Reset will increase slice count due to use of real FFs and instead of SRLs  en=off  latency=3  reg_retiming=off  dbl_ovrd=off  block_type=delay
  F1 : xbsIndex_r4/Constant  const=1023000  gui_display_data_type=Fixed-point  arith_type=Signed (2's comp)  n_bits=32  bin_pt=8  preci_type=Single  exp_width=8  frac_width=24  explicit_period=on  period=1/16367600  equ=P=C  opselect=C  inp2=PCIN>>17  opr=+  inp1=P  carry=CIN  dbl_ovrd=off  block_type=constant
  FilteredDLL : Scope
  FilteredDLLDiscriminator : xbsIndex_r4/Gateway Out  inherit_from_input=off  hdl_port=on  rows=1  columns=1  UseAsDAC=off  DACChannel='1'  interface=None  automatic_assignment=on  address_offset=hex2dec('00')  intf_name=''  intf_description=''  timing_constraint=None  locs_specified=off  LOCs={}  io_standard={}  block_type=gatewayout
  I2 : xbsIndex_r4/CMult  const=0.014317  gui_display_data_type=Fixed-point  const_n_bits=20  const_bin_pt=15  float_type=Single  exp_bits=8  fraction_bits=24  en=off  latency=2  precision=Full  arith_type="Signed  (2's comp)"  n_bits=16  bin_pt=14  quantization=Truncate  overflow=Wrap  use_behavioral_HDL=off  mem_type=Distributed RAM  pipeline=off  dbl_ovrd=off  block_type=cmult
  Out1 : Outport
  wires:
  F1/1 -> AddSub7/1
  en/1 -> Delay8/1, Delay5/2
  AddSub2/1 -> D1/1
  error/1 -> Delay5/1, I2/1, AddSub2/1
  Delay8/1 -> Delay7/2
  Delay7/1 -> AddSub6/1
  Delay5/1 -> AddSub2/2
  D1/1 -> AddSub5/1
  AddSub5/1 -> AddSub6/2
  I2/1 -> AddSub5/2
  AddSub7/1 -> D2/1
  D2/1 -> Out1/1
  AddSub6/1 -> FilteredDLLDiscriminator/1, AddSub7/2, Delay7/1
  FilteredDLLDiscriminator/1 -> FilteredDLL/1

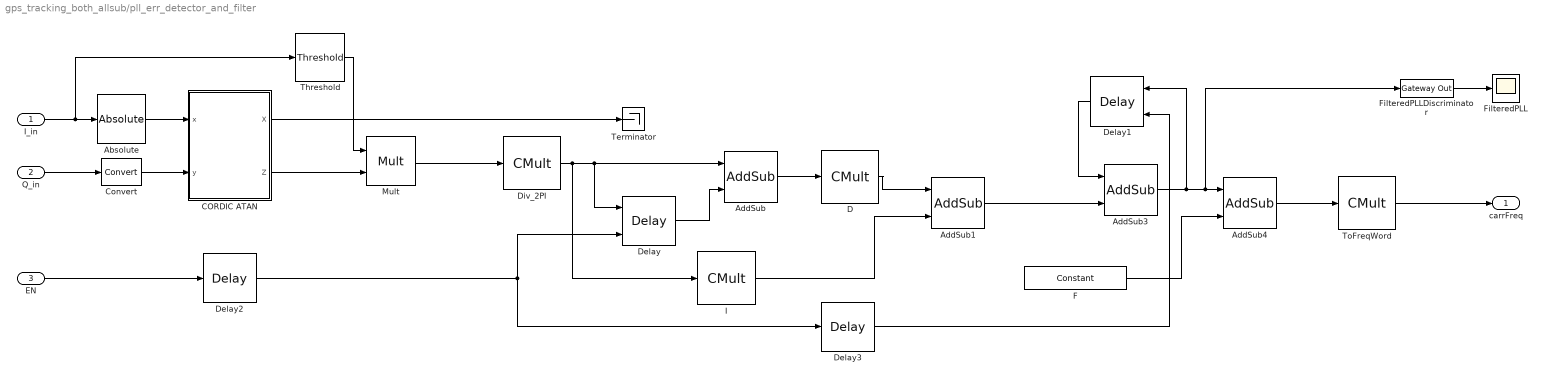
== system gps_tracking_both_allsub/pll_err_detector_and_filter ==
  I_in : Inport
  Q_in : Inport  Port=2
  EN : Inport  Port=3
  " FilteredPLLDiscriminator" : xbsIndex_r4/Gateway Out  inherit_from_input=off  hdl_port=on  rows=1  columns=1  UseAsDAC=off  DACChannel='1'  interface=None  automatic_assignment=on  address_offset=hex2dec('00')  intf_name=''  intf_description=''  timing_constraint=None  locs_specified=off  LOCs={}  io_standard={}  block_type=gatewayout
  Absolute : xbsIndex_r4/Absolute  precision=User Defined  arith_type="Signed  (2's comp)"  n_bits=30  bin_pt=14  quantization=Truncate  overflow=Flag as error  en=off  latency=1  dbl_ovrd=off  block_type=abs
  AddSub : xbsIndex_r4/AddSub  mode=Subtraction  use_carryin=off  use_carryout=off  en=off  latency=1  precision=Full  arith_type="Signed  (2's comp)"  n_bits=16  bin_pt=15  quantization=Truncate  overflow=Wrap  use_behavioral_HDL=off  hw_selection=Fabric  pipelined=off  dbl_ovrd=off  block_type=addsub
  AddSub1 : xbsIndex_r4/AddSub  mode=Addition  use_carryin=off  use_carryout=off  en=off  latency=1  precision=Full  arith_type="Signed  (2's comp)"  n_bits=16  bin_pt=15  quantization=Truncate  overflow=Wrap  use_behavioral_HDL=off  hw_selection=Fabric  pipelined=off  dbl_ovrd=off  block_type=addsub
  AddSub3 : xbsIndex_r4/AddSub  mode=Addition  use_carryin=off  use_carryout=off  en=off  latency=1  precision=User Defined  arith_type="Signed  (2's comp)"  n_bits=32  bin_pt=15  quantization=Truncate  overflow=Flag as error  use_behavioral_HDL=off  hw_selection=Fabric  pipelined=off  dbl_ovrd=off  block_type=addsub
  AddSub4 : xbsIndex_r4/AddSub  mode=Addition  use_carryin=off  use_carryout=off  en=off  latency=1  precision=Full  arith_type="Signed  (2's comp)"  n_bits=16  bin_pt=15  quantization=Truncate  overflow=Wrap  use_behavioral_HDL=off  hw_selection=Fabric  pipelined=off  dbl_ovrd=off  block_type=addsub
  CORDIC ATAN : Subsystem  mask(Xilinx CORDIC ATAN){stages=7, pe_nbits=30, pe_binpt=14, pipeline_x=ones(1,8), prev_stages=7, pipeline=[1  1  1  1  1  1  1]}
      mask prompts: stages "Number of Processing Elements (integer value starting from 1)"; pe_nbits "X, Y Data Width"; pe_binpt "X, Y Binary Point Position"; pipeline_x "Latency for each Processing Element [1 0 0 1]"; prev_stages "Previous Number of Stages"; pipeline "Previous Pipeline Values"
      mask help: A parallel implementation, circular vectoring mode CORDIC processor for performing rectangular-to-polar conversion. The number of iteration stages (and resultant output accuracy) and the processor arithmetic precision are controlled by the mask customization.
      mask init:
      | [bg,fg] = xlcmap('XBlock',0);
      | iPos = get_param(gcb,'Position');
      | iWidth=iPos(3)-iPos(1); iHeight=iPos(4)-iPos(2);
      | iCx=iWidth/2;
      | iCy=iHeight/2;
      | [logoX, logoY] = xlogo(iPos);
      | sav_gcb=gcb;
      | stages = round(sum(abs(stages)));
      | if (stages == 0)
      | 	stages = prev_stages;
      | end
      | x = zeros(1,stages);
      | pipe_size = max(size(pipeline_x));
      | if pipe_size >= stages
      | 	x(1,1:stages) = pipeline_x(1,1:stages);
      | else
      | 	x(1,1:pipe_size) = pipeline_x(1,1:pipe_size);
      | end
      | 
      | if (stages ~=prev_stages)
      | 	pipeline=x;
      | 	cordic_pe = find_system(gcb, 'lookUnderMasks', 'all', 'FollowLinks','on','masktype', 'CORDIC parallel PE');
      |     
      |   a=find_system(cordic_pe{1}, 'lookUnderMasks', 'all', 'FollowLinks','on','masktype', 'CORDIC iteration PE');
      |   for i= 2:length(a)
      |     for j=1:3
      | 	  delete_line(cordic_pe{1}, ['CORDIC PE' int2str(i-1) '/' int2str(j)], ['CORDIC PE' int2str(i) '/' int2str(j)]);
      |     end
      |   end
      |     if length(a)>0,
      |       delete_line(cordic_pe{1}, 'x/1', 'CORDIC PE1/1');
      |       delete_line(cordic_pe{1}, 'y/1', 'CORDIC PE1/2');
      |       delete_line(cordic_pe{1}, 'z/1', 'CORDIC PE1/3');
      |       delete_line(cordic_pe{1}, ['CORDIC PE' int2str(length(a)) '/1'],'X/1');
      |       delete_line(cordic_pe{1}, ['CORDIC PE' int2str(length(a)) '/2'],'Terminator/1');
      |       delete_line(cordic_pe{1}, ['CORDIC PE' int2str(length(a)) '/3'],'Z/1');
      |     elseif length(a)==0
      |       temp_port=get_param([cordic_pe{1} '/x'],'porthandles');
      |       temp_line=get_param(temp_port.Outport,'line');
      |       if temp_line>=0  delete_line(temp_line); end
      |       temp_port=get_param([cordic_pe{1} '/y'],'porthandles');
      |       temp_line=get_param(temp_port.Outport,'line');
      |       if temp_line>=0  delete_line(temp_line); end
      |       temp_port=get_param([cordic_pe{1} '/z'],'porthandles');
      |       temp_line=get_param(temp_port.Outport,'line');
      |       if temp_line>=0  delete_line(temp_line); end
      |     end
      | 
      |     for i=2:length(a)
      |       delete_block(a{i});
      |     end
      |     for i=2:stages,
      |         add_block([cordic_pe{1} '/CORDIC PE1'], [cordic_pe{1} '/CORDIC PE' int2str(i)], 'ii', int2str(i-1),'pe_nbits', 'pe_nbits','pe_binpt', 'pe_binpt','pipeline',['pipeline(1,' int2str(i) ')'],'position',[150+(i-1)*125, 70, 205+(i-1)*125, 130]);
      |     end
      | 
      |     for i= 2:stages,
      |       for j=1:3
      | 		add_line(cordic_pe{1}, ['CORDIC PE' int2str(i-1) '/' int2str(j)], ['CORDIC PE' int2str(i) '/' int2str(j)], 'autorouting', 'on');
      |       end
      |     end
      | 
      |     if stages==0
      |       add_line(cordic_pe{1}, 'x/1', 'X/1', 'autorouting', 'on');
      |       add_line(cordic_pe{1}, 'y/1', 'Terminator/1', 'autorouting', 'on');
      |       add_line(cordic_pe{1}, 'z/1', 'Z/1', 'autorouting', 'on');
      |     elseif stages>0
      |       add_line(cordic_pe{1}, 'x/1', 'CORDIC PE1/1', 'autorouting', 'on');
      |       add_line(cordic_pe{1}, 'y/1', 'CORDIC PE1/2', 'autorouting', 'on');
      |       add_line(cordic_pe{1}, 'z/1', 'CORDIC PE1/3', 'autorouting', 'on');
      | 
      |       set_param([cordic_pe{1} '/' 'X'], 'Position', [150+stages*125, 72, 180+stages*125, 86]);
      |       set_param([cordic_pe{1} '/' 'Terminator'], 'Position', [210+stages*125, 92, 225+stages*125, 108]);
      |       set_param([cordic_pe{1} '/' 'Z'], 'Position', [240+stages*125, 113, 270+stages*125, 127]);
      | 
      |       add_line(cordic_pe{1}, ['CORDIC PE' int2str(stages) '/1'], 'X/1', 'autorouting', 'on');
      |       add_line(cordic_pe{1}, ['CORDIC PE' int2str(stages) '/2'], 'Terminator/1', 'autorouting', 'on');
      |       add_line(cordic_pe{1}, ['CORDIC PE' int2str(stages) '/3'],'Z/1', 'autorouting', 'on');
      | 
      |       % force a "compile" of the constituent constant blocks to
      |       % workaround a data propagation problem
      |       find_system(cordic_pe{1}, 'lookUnderMasks', 'all', 'FollowLinks', 'on', 'MaskType','Xilinx Constant Block');
      |   end
      | 	set_param(sav_gcb, 'prev_stages', int2str(stages));
      | 	set_param(sav_gcb, 'pipeline', [ '[' int2str(x) ']']);
      | else
      | 	if (sum(pipeline~=x))
      | 		set_param(gcb, 'pipeline', [ '[' int2str(x) ']']);
      | 	end
      | end
      | str = sprintf('-%d',sum(x) + 3);
      settings: CopyFcn=set_param(gcb, 'MaskSelfModifiable', 'on', 'LinkStatus', 'none');
      mask Help: eval('');xlDoc('-book','sysgen','-topic','CORDIC_ATAN');
      mask Display:
      | patch([0 iWidth iWidth 0],[0 0 iHeight iHeight] , bg);
      | patch(logoX,logoY , fg);
      | text(iCx-6,iCy,'z');
      | text(iCx,iCy+4,str);
      | port_label('input',1,'x');
      | port_label('input',2,'y');
      | port_label('output',1,'mag');
      | port_label('output',2,'atan');
      | plot([0 0 iWidth iWidth 0], [0 iHeight iHeight 0 0]);
  Convert : xbsIndex_r4/Convert  gui_display_data_type=Fixed-point  arith_type="Signed  (2's comp)"  n_bits=30  bin_pt=14  float_type=Single  exp_bits=8  fraction_bits=24  quantization=Truncate  overflow=Wrap  en=off  latency=1  pipeline=off  dbl_ovrd=off  block_type=convert
  D : xbsIndex_r4/CMult  const=264.864865  gui_display_data_type=Fixed-point  const_n_bits=25  const_bin_pt=15  float_type=Single  exp_bits=8  fraction_bits=24  en=off  latency=1  precision=Full  arith_type="Signed  (2's comp)"  n_bits=16  bin_pt=14  quantization=Truncate  overflow=Wrap  use_behavioral_HDL=off  mem_type=Distributed RAM  pipeline=off  dbl_ovrd=off  block_type=cmult
  Delay : xbsIndex_r4/Delay  rst=off  infoeditControl=Selection of Reset will increase slice count due to use of real FFs and instead of SRLs  en=on  latency=1  reg_retiming=off  dbl_ovrd=off  block_type=delay
  Delay1 : xbsIndex_r4/Delay  rst=off  infoeditControl=Selection of Reset will increase slice count due to use of real FFs and instead of SRLs  en=on  latency=1  reg_retiming=off  dbl_ovrd=off  block_type=delay
  Delay2 : xbsIndex_r4/Delay  rst=off  infoeditControl=Selection of Reset will increase slice count due to use of real FFs and instead of SRLs  en=off  latency=11  reg_retiming=off  dbl_ovrd=off  block_type=delay
  Delay3 : xbsIndex_r4/Delay  rst=off  infoeditControl=Selection of Reset will increase slice count due to use of real FFs and instead of SRLs  en=off  latency=3  reg_retiming=off  dbl_ovrd=off  block_type=delay
  Div_2PI : xbsIndex_r4/CMult  const=1/2/pi  gui_display_data_type=Fixed-point  const_n_bits=32  const_bin_pt=32  float_type=Single  exp_bits=8  fraction_bits=24  en=off  latency=1  precision=User Defined  arith_type="Signed  (2's comp)"  n_bits=16  bin_pt=15  quantization=Truncate  overflow=Flag as error  use_behavioral_HDL=off  mem_type=Distributed RAM  pipeline=off  dbl_ovrd=off  block_type=cmult
  F : xbsIndex_r4/Constant  const=4.128433706474304e+06  gui_display_data_type=Fixed-point  arith_type=Signed (2's comp)  n_bits=32  bin_pt=8  preci_type=Single  exp_width=8  frac_width=24  explicit_period=on  period=1/16367600  equ=P=C  opselect=C  inp2=PCIN>>17  opr=+  inp1=P  carry=CIN  dbl_ovrd=off  block_type=constant
  FilteredPLL : Scope
  I : xbsIndex_r4/CMult  const=8.948137  gui_display_data_type=Fixed-point  const_n_bits=20  const_bin_pt=15  float_type=Single  exp_bits=8  fraction_bits=24  en=off  latency=2  precision=Full  arith_type="Signed  (2's comp)"  n_bits=16  bin_pt=14  quantization=Truncate  overflow=Wrap  use_behavioral_HDL=off  mem_type=Distributed RAM  pipeline=off  dbl_ovrd=off  block_type=cmult
  Mult : xbsIndex_r4/Mult  precision=Full  arith_type="Signed  (2's comp)"  n_bits=16  bin_pt=14  quantization=Truncate  overflow=Wrap  en=off  latency=0  use_behavioral_HDL=off  opt=Speed  use_embedded=on  optimum_pipeline=off  pipeline=on  dbl_ovrd=off  use_rpm=on  placement_style=Triangular  block_type=mult
  Terminator : Terminator
  Threshold : xbsIndex_r4/Threshold  en=off  latency=11  dbl_ovrd=off  block_type=sgn
      settings: infoedit="Presents -1 as output if input is negative; otherwise presents 1.  Output is a two bit signed number."
  ToFreqWord : xbsIndex_r4/CMult  const=6.1096312226594e-08  gui_display_data_type=Fixed-point  const_n_bits=48  const_bin_pt=48  float_type=Single  exp_bits=8  fraction_bits=24  en=off  latency=1  precision=User Defined  arith_type=Unsigned  n_bits=24  bin_pt=24  quantization=Truncate  overflow=Flag as error  use_behavioral_HDL=off  mem_type=Distributed RAM  pipeline=off  dbl_ovrd=off  block_type=cmult
  carrFreq : Outport
  wires:
  ToFreqWord/1 -> carrFreq/1
  F/1 -> AddSub4/2
  AddSub1/1 -> AddSub3/2
  Delay2/1 -> Delay3/1, Delay/2
  AddSub/1 -> D/1
  D/1 -> AddSub1/1
  CORDIC ATAN/2(Z) -> Mult/2
  Mult/1 -> Div_2PI/1
  AddSub4/1 -> ToFreqWord/1
  Threshold/1 -> Mult/1
  Q_in/1 -> Convert/1
  Delay3/1 -> Delay1/2
  I_in/1 -> Absolute/1, Threshold/1
  Delay1/1 -> AddSub3/1
  AddSub3/1 -> " FilteredPLLDiscriminator"/1, AddSub4/1, Delay1/1
  Absolute/1 -> CORDIC ATAN/1(x)
  EN/1 -> Delay2/1
  I/1 -> AddSub1/2
  Div_2PI/1 -> I/1, AddSub/1, Delay/1
  Delay/1 -> AddSub/2
  CORDIC ATAN/1(X) -> Terminator/1
  Convert/1 -> CORDIC ATAN/2(y)
  " FilteredPLLDiscriminator"/1 -> FilteredPLL/1

== system gps_tracking_both_allsub/pll_err_detector_and_filter/CORDIC ATAN ==
  note: The CORDIC algorithm is implemented in 3 steps.
      |
      | Step 1: Coarse Angle Rotation.  The algorithm converges only for angles between -pi/2 and pi/2, so if x < zero, the input vector is reflected
      | to the 1st or 3rd quadrant by making the x-coordinate non-negative.
      |
      | Step 2: Fine Angle Rotation.  For rectangular-to-polar conversion, the resulting vector is rotated through progressively smaller angles, such that y goes
      | to zero. In the i-th stage, the angular rotation is by either +/- atan(1/2^i), depending on whether or not its input y is less than or greater than zero.
      |
      | Step 3: Angle Correction. If there was a reflection applied in Step 1, this step applies the appropriate angle correction by subtracting it from +/- pi.
  x : Inport
  y : Inport  Port=2
  CORDIC Pipe Balance : xbsIndex_r4/Delay  rst=off  infoeditControl=Selection of Reset will increase slice count due to use of real FFs and instead of SRLs  en=off  latency=sum(pipeline)  reg_retiming=off  dbl_ovrd=off  block_type=delay
      settings: infoedit="Delay line having  configurable length.<P><P>Hardware notes: A delay line is a chain, each link of which is an SRL16 followed by a flip-flop. If register retiming is enabled, the delay line is a chain of flip-flops."  xl_area=[0, 0, 0, 0, 0, 0, 0]  block_version=VER_STRING_GOES_HERE
  CORDIC Pipe Balance1 : xbsIndex_r4/Delay  rst=off  infoeditControl=Selection of Reset will increase slice count due to use of real FFs and instead of SRLs  en=off  latency=sum(pipeline)+1  reg_retiming=off  dbl_ovrd=off  block_type=delay
      settings: infoedit="Delay line having  configurable length.<P><P>Hardware notes: A delay line is a chain, each link of which is an SRL16 followed by a flip-flop. If register retiming is enabled, the delay line is a chain of flip-flops."  xl_area=[0, 0, 0, 0, 0, 0, 0]  block_version=VER_STRING_GOES_HERE
  CORDIC Pipe Balance2 : xbsIndex_r4/Delay  rst=off  infoeditControl=Selection of Reset will increase slice count due to use of real FFs and instead of SRLs  en=off  latency=1  reg_retiming=off  dbl_ovrd=off  block_type=delay
      settings: infoedit="Delay line having  configurable length.<P><P>Hardware notes: A delay line is a chain, each link of which is an SRL16 followed by a flip-flop. If register retiming is enabled, the delay line is a chain of flip-flops."  xl_area=[0, 0, 0, 0, 0, 0, 0]  block_version=VER_STRING_GOES_HERE
  CORDIC Fine Angle PE : Subsystem  mask(CORDIC parallel PE){}
      mask init:
      | [bg,fg] = xlcmap('XBlock',0);
      | iPos = get_param(gcb,'Position');
      | iWidth=iPos(3)-iPos(1); iHeight=iPos(4)-iPos(2);
      | iCx=iWidth/2;
      | iCy=iHeight/2;
      | [logoX, logoY] = xlogo(iPos);
      mask Display:
      | patch([0 iWidth iWidth 0],[0 0 iHeight iHeight] , bg);
      | patch(logoX,logoY , fg);
      | port_label('input',1,'x');
      | port_label('input',2,'y');
      | port_label('input',3,'z');
      | port_label('output',1,'X');
      | port_label('output',2,'Z');
      | plot([0 0 iWidth iWidth 0], [0 iHeight iHeight 0 0]);
  Constant : xbsIndex_r4/Constant  const=0  gui_display_data_type=Fixed-point  arith_type=Signed (2's comp)  n_bits=pe_nbits  bin_pt=pe_binpt  preci_type=Single  exp_width=8  frac_width=24  explicit_period=off  period=1  equ=P=C  opselect=C  inp2=PCIN>>17  opr=+  inp1=P  carry=CIN  dbl_ovrd=off  block_type=constant
      settings: block_version=VER_STRING_GOES_HERE
  Quadrant Correct : Subsystem
      mask init:
      | [bg,fg] = xlcmap('XBlock',0);
      | iPos = get_param(gcb,'Position');
      | iWidth=iPos(3)-iPos(1); iHeight=iPos(4)-iPos(2);
      | iCx=iWidth/2;
      | iCy=iHeight/2;
      | [logoX, logoY] = xlogo(iPos);
      mask Display:
      | patch([0 iWidth iWidth 0],[0 0 iHeight iHeight] , bg);
      | patch(logoX,logoY , fg);
      | port_label('input',1,'Z in');
      | port_label('input',2,'sgn(y)');
      | port_label('input',3,'sgn(x)');
      | port_label('output',1,'Z');
      | plot([0 0 iWidth iWidth 0], [0 iHeight iHeight 0 0]);
  Quadrant Map : Subsystem
      mask init:
      | [bg,fg] = xlcmap('XBlock',0);
      | iPos = get_param(gcb,'Position');
      | iWidth=iPos(3)-iPos(1); iHeight=iPos(4)-iPos(2);
      | iCx=iWidth/2;
      | iCy=iHeight/2;
      | [logoX, logoY] = xlogo(iPos);
      mask Display:
      | patch([0 iWidth iWidth 0],[0 0 iHeight iHeight] , bg);
      | patch(logoX,logoY , fg);
      | port_label('input',1,'x');
      | port_label('input',2,'y');
      | port_label('output',1,'X');
      | port_label('output',2,'Y');
      | port_label('output',3,'sgn(y)');
      | port_label('output',4,'sgn(x)');
      | plot([0 0 iWidth iWidth 0], [0 iHeight iHeight 0 0]);
  X : Outport
  Z : Outport  Port=2
  wires:
  CORDIC Pipe Balance2/1 -> X/1
  CORDIC Fine Angle PE/1(X) -> CORDIC Pipe Balance2/1
  Quadrant Correct/1(Z) -> Z/1
  CORDIC Fine Angle PE/2(Z) -> Quadrant Correct/1(Z IN)
  CORDIC Pipe Balance1/1 -> Quadrant Correct/3(Z MUX SEL)
  CORDIC Pipe Balance/1 -> Quadrant Correct/2(PI_ addsub)
  Quadrant Map/4(sign(x)) -> CORDIC Pipe Balance1/1
  Quadrant Map/3(sign(y)) -> CORDIC Pipe Balance/1
  y/1 -> Quadrant Map/2(y)
  x/1 -> Quadrant Map/1(x)
  Quadrant Map/2(Y) -> CORDIC Fine Angle PE/2(y)
  Quadrant Map/1(X) -> CORDIC Fine Angle PE/1(x)
  Constant/1 -> CORDIC Fine Angle PE/3(z)
